simulink model "Coletor_Admissao"  (R2025b)
settings: Solver=VariableStepAuto  StartTime=0.0  StopTime=10.0  RelTol=1e-3
undefined symbols (not defined in the file): R, V
settings Model: Creator=ivomu  LastModifiedBy=ivomu

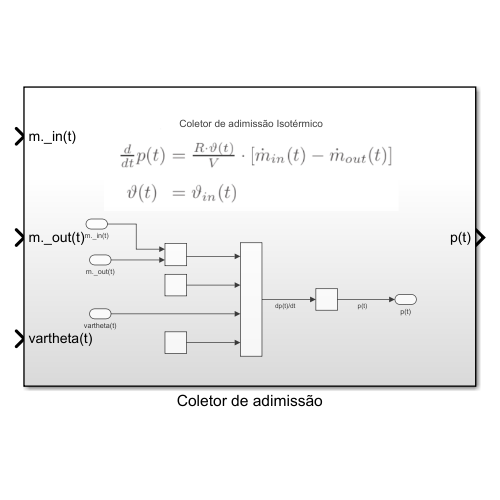
[thumbnail: Simulink's stored preview of the top-level diagram]
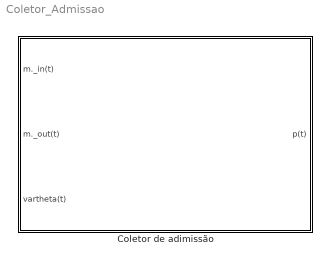
== system Coletor_Admissao ==
  Coletor de adimissão : Subsystem

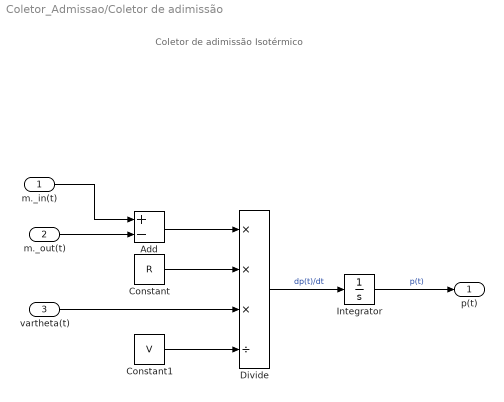
== system Coletor_Admissao/Coletor de adimissão ==
  note: Coletor de adimissão Isotérmico
  m._in(t) : Inport
  m._out(t) : Inport  Port=2
  vartheta(t) : Inport  Port=3
  Add : Sum  Inputs=+-
  Constant : Constant  Value=R
  Constant1 : Constant  Value=V
  Divide : Product  Inputs=***/
  Integrator : Integrator
  p(t) : Outport
  wires:
  Add/1 -> Divide/1
  Constant/1 -> Divide/2
  m._in(t)/1 -> Add/1
  Divide/1 -> Integrator/1  "dp(t)/dt"
  Constant1/1 -> Divide/4
  m._out(t)/1 -> Add/2
  Integrator/1 -> p(t)/1  "p(t)"
  vartheta(t)/1 -> Divide/3
